simulink model "speedgoat_test_SN5659_R2021b_IO107"  (R2021b)
settings: Solver=FixedStepDiscrete  StartTime=0.0  StopTime=inf  RelTol=1e-3
PreLoadFcn:
  | Ts_IO107 = 0.001;
  | Ts_IO107 = 0.001;
  | Ts_IO133 = 0.001
  | 
  | Ts_IO204 = 0.001;
  | 
  | 
  | Ts_IO503 = 0.01;
  | 
  | ts_IO612 = 1e-3;
  | Ts_IO682 = 0.005;
  | Ts_IO941 = 0.01;
InitFcn:
  | Ts_IO107 = 0.001;
  | Ts_IO107 = 0.001;
  | Ts_IO133 = 0.001
  | 
  | Ts_IO204 = 0.001;
  | 
  | 
  | Ts_IO503 = 0.01;
  | 
  | ts_IO612 = 1e-3;
  | Ts_IO682 = 0.005;
  | Ts_IO941 = 0.01;
StopFcn:
  | if isfile(['sdi_view_',bdroot,'.mldatx'])
  |  Simulink.sdi.clearPreferences();
  |  Simulink.sdi.view();
  |  pause(3);
  |  Simulink.sdi.loadView(['sdi_view_',bdroot,]);
  | end
libraries: speedgoatlib_IO107 x4, simulink x1
settings Model: Creator=yannick.orgas  LastModifiedBy=ACH
settings SolverCC: ConcurrentTasks=on  AlgebraicLoopSolver=TrustRegion  PositivePriorityOrder=on
settings DataIOCC: LimitDataPoints=on  SaveFormat=StructureWithTime
settings OptimizationCC: BlockReduction=off  OptimizeBlockIOStorage=off
settings DebuggingCC: TasksWithSamePriorityMsg=none  UnconnectedInputMsg=none  UnconnectedOutputMsg=none  UnconnectedLineMsg=none  SFMachineParentedDataDiag=warning
settings HardwareCC: ProdBitPerLong=64  ProdLongLongMode=on  ProdHWDeviceType=Intel->x86-64 (Linux 64)
settings RTWCC: Description=Simulink Real-Time  SystemTargetFile=slrealtime.tlc  TemplateMakefile=slrealtime_default_tmf  Toolchain=Simulink Real-Time Toolchain  BuildConfiguration=Faster Runs  CodeExecutionProfiling=on  TargetLang=C++
settings SimulinkRealTimeTargetCC: UseGCCFastMath=on

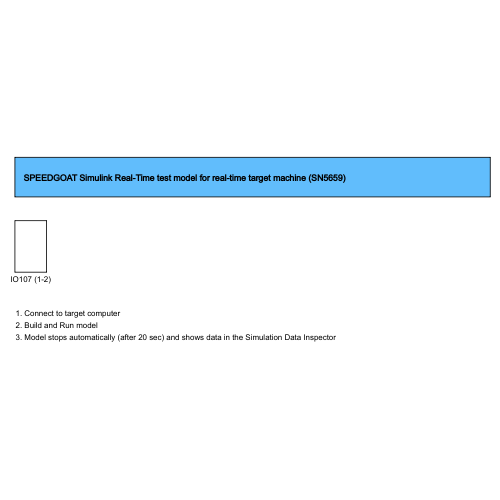
[thumbnail: Simulink's stored preview of the top-level diagram]
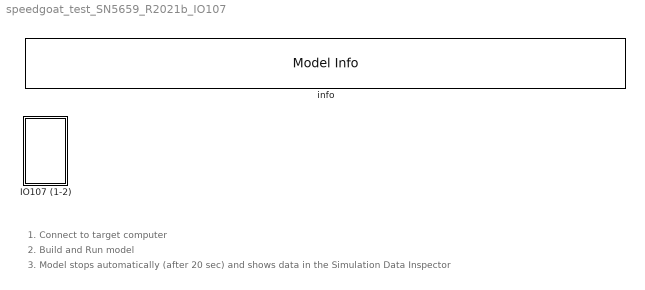
== system speedgoat_test_SN5659_R2021b_IO107 ==
  note: 1. Connect to target computer
  note: 2. Build and Run model
  note: 3. Model stops automatically (after 20 sec) and shows data in the Simulation Data Inspector
  IO107 (1-2) : Subsystem
  info : simulink/Model-Wide Utilities/Model Info  Frame=on  DisplayStringWithTags=SPEEDGOAT Simulink Real-Time test model for real-time target machine (SN5659)  HorizontalTextAlignment=Left  LeftAlignmentValue=0.02

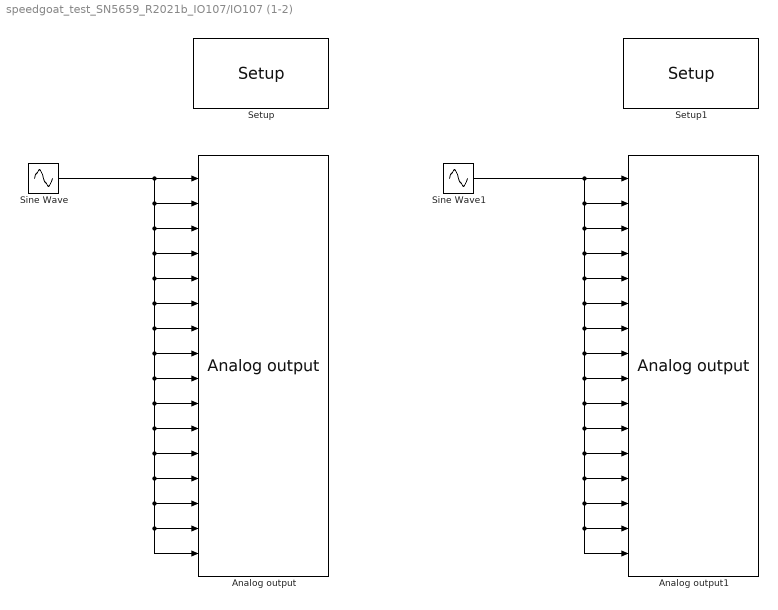
== system speedgoat_test_SN5659_R2021b_IO107/IO107 (1-2) ==
  Analog output : speedgoatlib_IO107/Analog output  id=1  ts=-1  index=[1 2 3 4 5 6 7 8 9 10 11 12 13 14 15 16]  channels=[1 2 3 4 5 6 7 8 9 10 11 12 13 14 15 16]  range=1  pciSlot=-1
      settings: SourceProductName=Simulink Real-Time: Speedgoat Library
  Analog output1 : speedgoatlib_IO107/Analog output  id=2  ts=-1  index=[1 2 3 4 5 6 7 8 9 10 11 12 13 14 15 16]  channels=[1 2 3 4 5 6 7 8 9 10 11 12 13 14 15 16]  range=1  pciSlot=-1
      settings: SourceProductName=Simulink Real-Time: Speedgoat Library
  Setup : speedgoatlib_IO107/Setup  group=Analog output setup  id=1  range=+-10V  triggerSignal=TTL  groundSense=off  cal=on  pciSlot=-1  daChannel=[1:16]  daInitValue=[0]  daReset=[1]
      settings: SourceProductName=Simulink Real-Time: Speedgoat Library
  Setup1 : speedgoatlib_IO107/Setup  group=Module setup  id=2  range=+-10V  triggerSignal=TTL  groundSense=off  cal=on  pciSlot=-1  daChannel=[1:16]  daInitValue=[0]  daReset=[1]
      settings: SourceProductName=Simulink Real-Time: Speedgoat Library
  Sine Wave : Sin  Amplitude=10  Frequency=2*pi*50  SampleTime=Ts_IO107
  Sine Wave1 : Sin  Amplitude=10  Frequency=2*pi*200  SampleTime=Ts_IO107
  wires:
  Sine Wave1/1 -> Analog output1/1, Analog output1/2, Analog output1/3, Analog output1/4, Analog output1/5, Analog output1/6, Analog output1/7, Analog output1/8, Analog output1/9, Analog output1/10, Analog output1/11, Analog output1/12, Analog output1/13, Analog output1/14, Analog output1/15, Analog output1/16
  Sine Wave/1 -> Analog output/1, Analog output/2, Analog output/3, Analog output/4, Analog output/5, Analog output/6, Analog output/7, Analog output/8, Analog output/9, Analog output/10, Analog output/11, Analog output/12, Analog output/13, Analog output/14, Analog output/15, Analog output/16
